simulink model "gm_carga_HDLGEN"  (R2018a)
settings: Solver=FixedStepDiscrete  StartTime=0.0  StopTime=.2  FixedStep=1e-4  RelTol=1e-3
InitFcn:
  | Hs = tf([520 0], [1.3801 104 100]);
  | Hz = c2d(Hs, 1e-4, 'impulse');
libraries: hdlmdlgenlib x2
settings Model: FPTRunName=Ranges(Double)  Creator=erich  LastModifiedBy=erich
settings DataIOCC: SaveOutput=off  SaveTime=off
settings OptimizationCC: BlockReduction=off  ConditionallyExecuteInputs=off  DefaultParameterBehavior=Inlined
settings DebuggingCC: AlgebraicLoopMsg=error  InheritedTsInSrcMsg=none  SingleTaskRateTransMsg=error  StrictBusMsg=ErrorOnBusTreatedAsVector
settings HardwareCC: ProdBitPerPointer=32  ProdBitPerSizeT=32  ProdBitPerPtrDiffT=32  ProdLargestAtomicFloat=None  ProdIntDivRoundTo=Undefined  ProdEndianess=Unspecified  ProdWordSize=32  ProdHWDeviceType=ASIC/FPGA->ASIC/FPGA  ProdEqTarget=off
settings CodeAppCC: StateflowObjectComments=on
settings GRTTargetCC: TargetLangStandard=C89/C90 (ANSI)

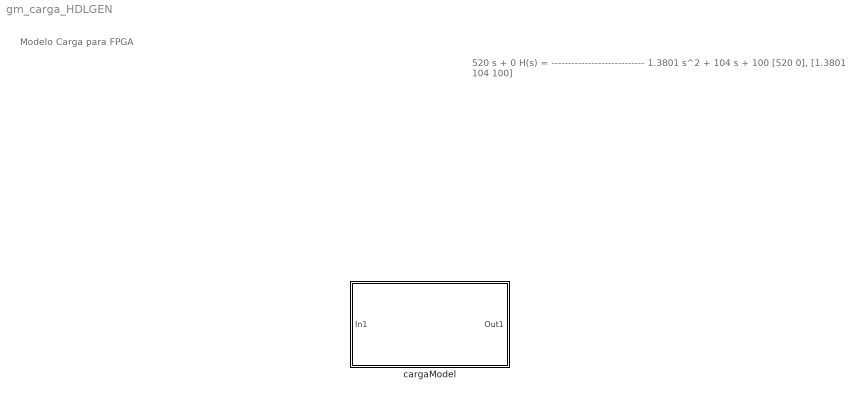
== system gm_carga_HDLGEN ==
  note: Modelo Carga
      | para FPGA
  note: 520 s + 0
      | H(s) = ----------------------------
      | 1.3801 s^2 + 104 s + 100
      |
      | [520 0], [1.3801 104 100]
  cargaModel : Subsystem

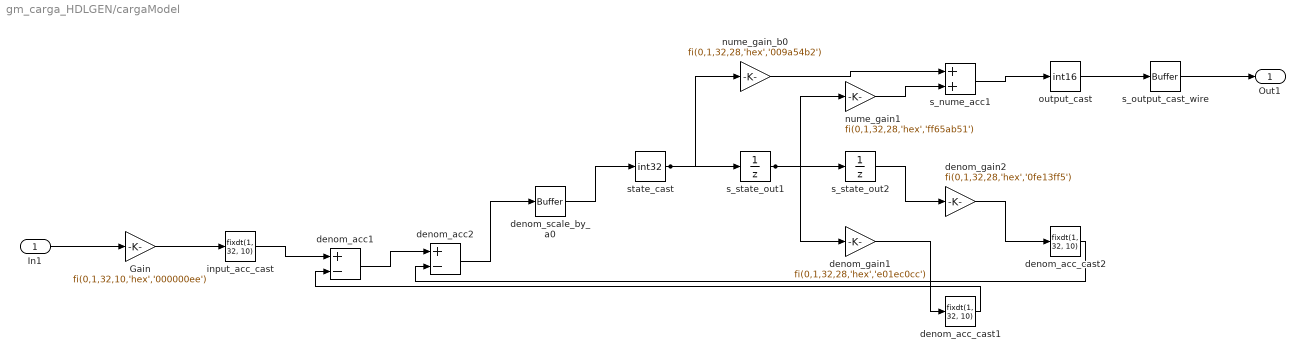
== system gm_carga_HDLGEN/cargaModel ==
  In1 : Inport  OutDataTypeStr=int16  PortDimensions=1
  Gain : Gain  Gain=fi(0,1,32,10,'hex','000000ee')  ParamDataTypeStr=fixdt(1, 32, 10)  OutDataTypeStr=fixdt(1, 48, 10)
  denom_acc1 : Sum  Inputs=+-  AccumDataTypeStr=fixdt(1, 32, 10)  OutDataTypeStr=fixdt(1, 32, 10)  RndMeth=Round
  denom_acc2 : Sum  Inputs=+-  AccumDataTypeStr=fixdt(1, 32, 10)  OutDataTypeStr=fixdt(1, 32, 10)  RndMeth=Round
  denom_acc_cast1 : DataTypeConversion  OutDataTypeStr=fixdt(1, 32, 10)  RndMeth=Round
  denom_acc_cast2 : DataTypeConversion  OutDataTypeStr=fixdt(1, 32, 10)  RndMeth=Round
  denom_gain1 : Gain  Gain=fi(0,1,32,28,'hex','e01ec0cc')  ParamDataTypeStr=fixdt(1, 32, 28)  OutDataTypeStr=fixdt(1, 32, 10)  RndMeth=Round
  denom_gain2 : Gain  Gain=fi(0,1,32,28,'hex','0fe13ff5')  ParamDataTypeStr=fixdt(1, 32, 28)  OutDataTypeStr=fixdt(1, 32, 10)  RndMeth=Round
  denom_scale_by_a0 : hdlmdlgenlib/Buffer
      settings: SourceProductName=HDL Coder  SourceProductBaseCode=HD
  input_acc_cast : DataTypeConversion  OutDataTypeStr=fixdt(1, 32, 10)  RndMeth=Round
  nume_gain1 : Gain  Gain=fi(0,1,32,28,'hex','ff65ab51')  ParamDataTypeStr=fixdt(1, 32, 28)  OutDataTypeStr=fixdt(1, 32, 10)  RndMeth=Round
  nume_gain_b0 : Gain  Gain=fi(0,1,32,28,'hex','009a54b2')  ParamDataTypeStr=fixdt(1, 32, 28)  OutDataTypeStr=fixdt(1, 32, 10)  RndMeth=Round
  output_cast : DataTypeConversion  OutDataTypeStr=int16  RndMeth=Round
  s_nume_acc1 : Sum  OutDataTypeStr=fixdt(1, 32, 10)  RndMeth=Round
  s_output_cast_wire : hdlmdlgenlib/Buffer
      settings: SourceProductName=HDL Coder  SourceProductBaseCode=HD
  s_state_out1 : UnitDelay  InitialCondition=fi(0,1,32,0,'hex','00000000')
  s_state_out2 : UnitDelay  InitialCondition=fi(0,1,32,0,'hex','00000000')
  state_cast : DataTypeConversion  OutDataTypeStr=int32  RndMeth=Round
  Out1 : Outport  OutDataTypeStr=int16
  wires:
  In1/1 -> Gain/1
  s_output_cast_wire/1 -> Out1/1
  Gain/1 -> input_acc_cast/1
  input_acc_cast/1 -> denom_acc1/1
  denom_acc_cast1/1 -> denom_acc1/2
  denom_acc1/1 -> denom_acc2/1
  denom_acc_cast2/1 -> denom_acc2/2
  denom_acc2/1 -> denom_scale_by_a0/1
  denom_scale_by_a0/1 -> state_cast/1
  state_cast/1 -> nume_gain_b0/1, s_state_out1/1
  s_state_out1/1 -> nume_gain1/1, denom_gain1/1, s_state_out2/1
  s_state_out2/1 -> denom_gain2/1
  denom_gain1/1 -> denom_acc_cast1/1
  denom_gain2/1 -> denom_acc_cast2/1
  nume_gain_b0/1 -> s_nume_acc1/1
  nume_gain1/1 -> s_nume_acc1/2
  s_nume_acc1/1 -> output_cast/1
  output_cast/1 -> s_output_cast_wire/1
